simulink model "Pacemaker_OperatingModes"  (R2020a)
settings: Solver=FixedStepAuto  StartTime=0.0  StopTime=10.0  FixedStep=1e-3  RelTol=1e-3  EnableMultiTasking=on
undefined symbols (not defined in the file): D0, D1, D10, D11, D12, D13, D2, D3, D4, D5, D6, D7, D8, D9, PTA0, PTA1, PTA2, PTB23, PTB9, PTC16, PTC17, PTC2, PTC3, PTC4, PTD0, PTD1, PTD2, PTD3
libraries: frdmk64flib x14
settings Model: ExtModeTrigDuration=5  Creator=furqa  LastModifiedBy=furqa
settings OptimizationCC: EnhancedBackFolding=on  PassReuseOutputArgsAs=Individual arguments  ZeroExternalMemoryAtStartup=off  ZeroInternalMemoryAtStartup=off  MaxStackSize=64  OptimizeBlockOrder=speed  DifferentSizesBufferReuse=on  OptimizationCustomize=off  EfficientTunableParamExpr=on
settings DebuggingCC: ParameterTunabilityLossMsg=error
settings HardwareCC: ProdBitPerPointer=32  ProdBitPerSizeT=32  ProdBitPerPtrDiffT=32  ProdLargestAtomicInteger=Long  ProdLargestAtomicFloat=Double  ProdWordSize=32  ProdHWDeviceType=ARM Compatible->ARM Cortex
settings SFSimCC: MATLABDynamicMemAlloc=off
settings RTWCC: SystemTargetFile=ert.tlc  HardwareBoard=NXP FRDM-K64F  TemplateMakefile=ert_default_tmf  Toolchain=GNU Tools for ARM Embedded Processors
settings CodeAppCC: ForceParamTrailComments=on  IgnoreCustomStorageClasses=off  OperatorAnnotations=on  SimulinkDataObjDesc=on  SFDataObjDesc=on  InsertBlockDesc=on

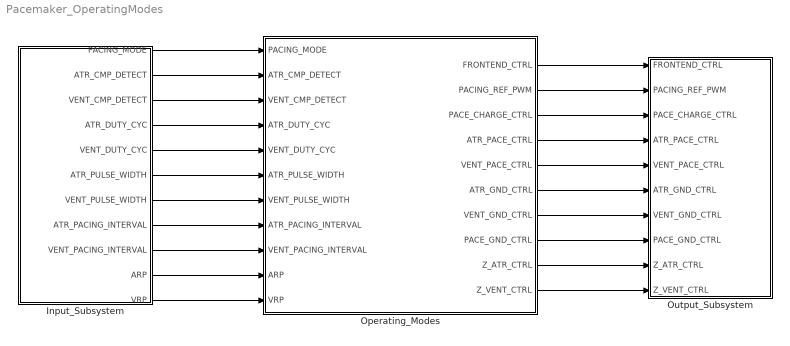
== system Pacemaker_OperatingModes ==
  Input_Subsystem : Subsystem
  Operating_Modes : Stateflow chart  TreatAsAtomicUnit=on
  Output_Subsystem : Subsystem
  wires:
  Input_Subsystem/1(PACING_MODE) -> Operating_Modes/1(PACING_MODE)
  Input_Subsystem/4(ATR_DUTY_CYC) -> Operating_Modes/4(ATR_DUTY_CYC)
  Input_Subsystem/5(VENT_DUTY_CYC) -> Operating_Modes/5(VENT_DUTY_CYC)
  Input_Subsystem/6("ATR_PULSE_WIDTH ") -> Operating_Modes/6(ATR_PULSE_WIDTH)
  Input_Subsystem/7("VENT_PULSE_WIDTH ") -> Operating_Modes/7(VENT_PULSE_WIDTH)
  Input_Subsystem/8("ATR_PACING_INTERVAL ") -> Operating_Modes/8(ATR_PACING_INTERVAL)
  Input_Subsystem/9("VENT_PACING_INTERVAL ") -> Operating_Modes/9(VENT_PACING_INTERVAL)
  Operating_Modes/1(FRONTEND_CTRL) -> Output_Subsystem/1(FRONTEND_CTRL)
  Operating_Modes/2(PACING_REF_PWM) -> Output_Subsystem/2(PACING_REF_PWM)
  Operating_Modes/3(PACE_CHARGE_CTRL) -> Output_Subsystem/3(PACE_CHARGE_CTRL)
  Operating_Modes/4(ATR_PACE_CTRL) -> Output_Subsystem/4(ATR_PACE_CTRL)
  Operating_Modes/5(VENT_PACE_CTRL) -> Output_Subsystem/5(VENT_PACE_CTRL)
  Operating_Modes/6(ATR_GND_CTRL) -> Output_Subsystem/6(ATR_GND_CTRL)
  Operating_Modes/7(VENT_GND_CTRL) -> Output_Subsystem/7(VENT_GND_CTRL)
  Operating_Modes/8(PACE_GND_CTRL) -> Output_Subsystem/8(PACE_GND_CTRL)
  Operating_Modes/9(Z_ATR_CTRL) -> Output_Subsystem/9(Z_ATR_CTRL)
  Operating_Modes/10(Z_VENT_CTRL) -> Output_Subsystem/10(Z_VENT_CTRL)
  Input_Subsystem/2(ATR_CMP_DETECT) -> Operating_Modes/2(ATR_CMP_DETECT)
  Input_Subsystem/3(VENT_CMP_DETECT) -> Operating_Modes/3(VENT_CMP_DETECT)
  Input_Subsystem/10(ARP) -> Operating_Modes/10(ARP)
  Input_Subsystem/11(VRP) -> Operating_Modes/11(VRP)

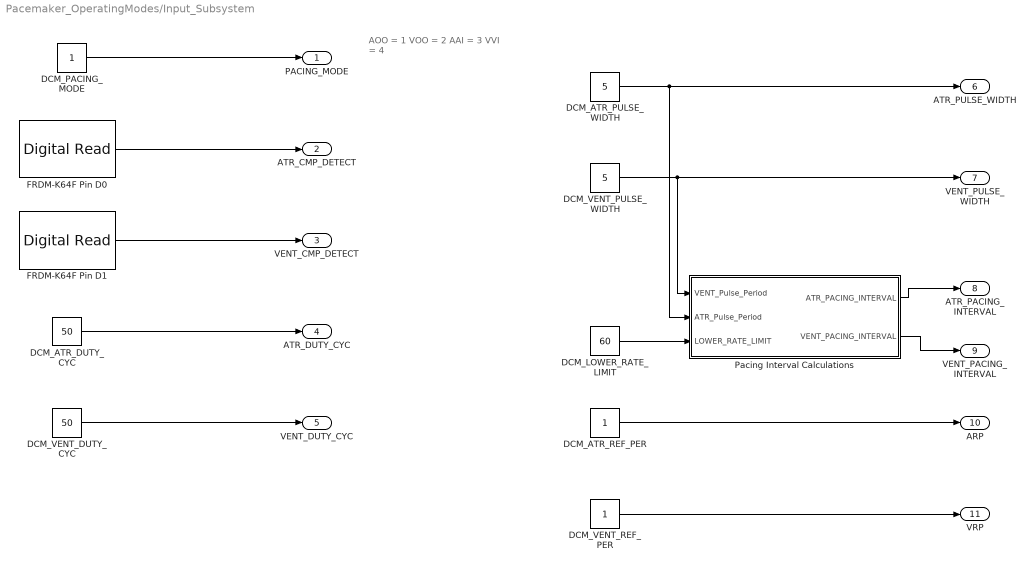
== system Pacemaker_OperatingModes/Input_Subsystem ==
  note: AOO = 1
      | VOO = 2
      | AAI = 3
      | VVI = 4
  DCM_ATR_DUTY_CYC : Constant  Value=50
  "DCM_ATR_PULSE_WIDTH " : Constant  Value=5
  DCM_ATR_REF_PER : Constant
  DCM_LOWER_RATE_LIMIT : Constant  Value=60
  DCM_PACING_MODE : Constant
  DCM_VENT_DUTY_CYC : Constant  Value=50
  "DCM_VENT_PULSE_WIDTH " : Constant  Value=5
  DCM_VENT_REF_PER : Constant
  FRDM-K64F Pin D0 : frdmk64flib/Digital Read  Whichpin=PTC16 (D0)  SampleTime=-1
  FRDM-K64F Pin D1 : frdmk64flib/Digital Read  Whichpin=PTC17 (D1)  SampleTime=-1
  Pacing Interval Calculations : Subsystem
  PACING_MODE : Outport
  ATR_CMP_DETECT : Outport  Port=2
  VENT_CMP_DETECT : Outport  Port=3
  ATR_DUTY_CYC : Outport  Port=4
  VENT_DUTY_CYC : Outport  Port=5
  "ATR_PULSE_WIDTH " : Outport  Port=6
  "VENT_PULSE_WIDTH " : Outport  Port=7
  "ATR_PACING_INTERVAL " : Outport  Port=8
  "VENT_PACING_INTERVAL " : Outport  Port=9
  ARP : Outport  Port=10
  VRP : Outport  Port=11
  wires:
  DCM_PACING_MODE/1 -> PACING_MODE/1
  FRDM-K64F Pin D0/1 -> ATR_CMP_DETECT/1
  FRDM-K64F Pin D1/1 -> VENT_CMP_DETECT/1
  DCM_ATR_DUTY_CYC/1 -> ATR_DUTY_CYC/1
  DCM_VENT_DUTY_CYC/1 -> VENT_DUTY_CYC/1
  "DCM_ATR_PULSE_WIDTH "/1 -> Pacing Interval Calculations/2(ATR_Pulse_Period), "ATR_PULSE_WIDTH "/1
  "DCM_VENT_PULSE_WIDTH "/1 -> "VENT_PULSE_WIDTH "/1, Pacing Interval Calculations/1(VENT_Pulse_Period)
  DCM_LOWER_RATE_LIMIT/1 -> Pacing Interval Calculations/3(LOWER_RATE_LIMIT)
  Pacing Interval Calculations/1(ATR_PACING_INTERVAL) -> "ATR_PACING_INTERVAL "/1
  Pacing Interval Calculations/2(VENT_PACING_INTERVAL) -> "VENT_PACING_INTERVAL "/1
  DCM_ATR_REF_PER/1 -> ARP/1
  DCM_VENT_REF_PER/1 -> VRP/1

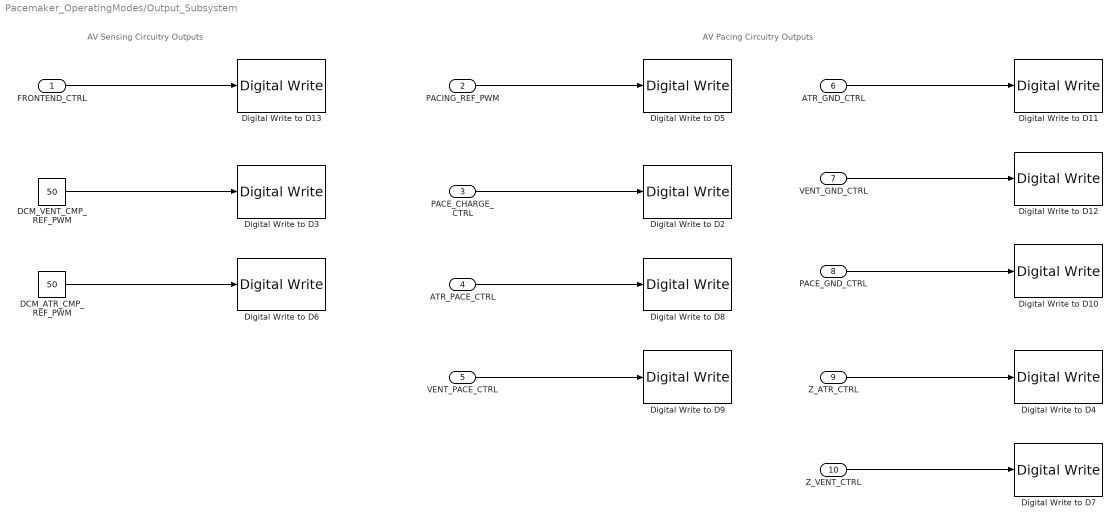
== system Pacemaker_OperatingModes/Output_Subsystem ==
  note: AV Pacing Circuitry Outputs
  note: AV Sensing Circuitry Outputs
  FRONTEND_CTRL : Inport
  PACING_REF_PWM : Inport  Port=2
  PACE_CHARGE_CTRL : Inport  Port=3
  ATR_PACE_CTRL : Inport  Port=4
  VENT_PACE_CTRL : Inport  Port=5
  ATR_GND_CTRL : Inport  Port=6
  VENT_GND_CTRL : Inport  Port=7
  PACE_GND_CTRL : Inport  Port=8
  Z_ATR_CTRL : Inport  Port=9
  Z_VENT_CTRL : Inport  Port=10
  DCM_ATR_CMP_REF_PWM : Constant  Value=50
  DCM_VENT_CMP_REF_PWM : Constant  Value=50
  Digital Write to D10 : frdmk64flib/Digital Write  Whichpin=PTD0 (D10)
  Digital Write to D11 : frdmk64flib/Digital Write  Whichpin=PTD2 (D11)
  Digital Write to D12 : frdmk64flib/Digital Write  Whichpin=PTD3 (D12)
  Digital Write to D13 : frdmk64flib/Digital Write  Whichpin=PTD1 (D13)
  Digital Write to D2 : frdmk64flib/Digital Write  Whichpin=PTB9 (D2)
  Digital Write to D3 : frdmk64flib/Digital Write  Whichpin=PTA1 (D3)
  Digital Write to D4 : frdmk64flib/Digital Write  Whichpin=PTB23 (D4)
  Digital Write to D5 : frdmk64flib/Digital Write  Whichpin=PTA2 (D5)
  Digital Write to D6 : frdmk64flib/Digital Write  Whichpin=PTC2 (D6)
  Digital Write to D7 : frdmk64flib/Digital Write  Whichpin=PTC3 (D7)
  Digital Write to D8 : frdmk64flib/Digital Write  Whichpin=PTA0 (D8)
  Digital Write to D9 : frdmk64flib/Digital Write  Whichpin=PTC4 (D9)
  wires:
  FRONTEND_CTRL/1 -> Digital Write to D13/1
  DCM_VENT_CMP_REF_PWM/1 -> Digital Write to D3/1
  DCM_ATR_CMP_REF_PWM/1 -> Digital Write to D6/1
  PACING_REF_PWM/1 -> Digital Write to D5/1
  PACE_CHARGE_CTRL/1 -> Digital Write to D2/1
  ATR_PACE_CTRL/1 -> Digital Write to D8/1
  VENT_GND_CTRL/1 -> Digital Write to D12/1
  VENT_PACE_CTRL/1 -> Digital Write to D9/1
  ATR_GND_CTRL/1 -> Digital Write to D11/1
  PACE_GND_CTRL/1 -> Digital Write to D10/1
  Z_ATR_CTRL/1 -> Digital Write to D4/1
  Z_VENT_CTRL/1 -> Digital Write to D7/1

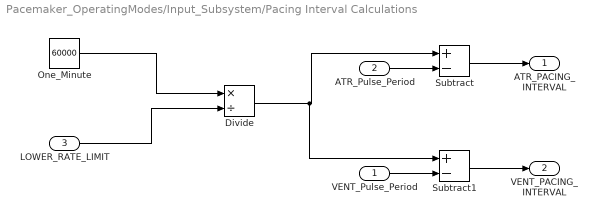
== system Pacemaker_OperatingModes/Input_Subsystem/Pacing Interval Calculations ==
  VENT_Pulse_Period : Inport
  ATR_Pulse_Period : Inport  Port=2
  LOWER_RATE_LIMIT : Inport  Port=3
  Divide : Product  Inputs=*/
  One_Minute : Constant  Value=60000
  Subtract : Sum  Inputs=+-
  Subtract1 : Sum  Inputs=+-
  ATR_PACING_INTERVAL : Outport
  VENT_PACING_INTERVAL : Outport  Port=2
  wires:
  One_Minute/1 -> Divide/1
  LOWER_RATE_LIMIT/1 -> Divide/2
  ATR_Pulse_Period/1 -> Subtract/2
  Subtract/1 -> ATR_PACING_INTERVAL/1
  VENT_Pulse_Period/1 -> Subtract1/2
  Divide/1 -> Subtract1/1, Subtract/1
  Subtract1/1 -> VENT_PACING_INTERVAL/1

== stateflow chart Pacemaker_OperatingModes/Operating_Modes ==
  state AOO
    state AOO_Pace_OFF
      during:
      ATR_PACE_CTRL = false
      VENT_PACE_CTRL = false
      PACING_REF_PWM = ATR_DUTY_CYC
      PACE_CHARGE_CTRL = true
      PACE_GND_CTRL = true
      Z_ATR_CTRL = false
      Z_VENT_CTRL = false
      ATR_GND_CTRL = true
      VENT_GND_CTRL = false
      FRONTEND_CTRL = false
    state AOO_Pace_ON
      during:
      PACE_CHARGE_CTRL = false
      PACE_GND_CTRL = true
      ATR_PACE_CTRL = true
      ATR_GND_CTRL = false
      Z_ATR_CTRL = false
      Z_VENT_CTRL = false
      VENT_GND_CTRL = false
      VENT_PACE_CTRL = false
      FRONTEND_CTRL = false
    (default) -> AOO_Pace_OFF
    AOO_Pace_OFF -> AOO_Pace_ON : after(ATR_PACING_INTERVAL, msec)
    AOO_Pace_ON -> AOO_Pace_OFF : after(ATR_PULSE_WIDTH, msec)
  state VVI
    state VVI_Pace_OFF
      during:
      ATR_PACE_CTRL = false
      VENT_PACE_CTRL = false
      PACING_REF_PWM =  VENT_DUTY_CYC
      PACE_CHARGE_CTRL = true
      PACE_GND_CTRL = true
      Z_ATR_CTRL = false
      Z_VENT_CTRL = false
      ATR_GND_CTRL = false
      VENT_GND_CTRL = true
      FRONTEND_CTRL = true
    state VVI_Pace_SENSED
      during:
      ATR_PACE_CTRL = false
      VENT_PACE_CTRL = false
      PACE_CHARGE_CTRL = true
      PACE_GND_CTRL = true
      Z_ATR_CTRL = false
      Z_VENT_CTRL = false
      ATR_GND_CTRL = false
      VENT_GND_CTRL = true
      FRONTEND_CTRL = false
    state VVI_Pace_ON
      during:
      PACE_CHARGE_CTRL = false
      PACE_GND_CTRL = true
      ATR_PACE_CTRL = false
      ATR_GND_CTRL = false
      Z_ATR_CTRL = false
      Z_VENT_CTRL = false
      VENT_GND_CTRL = false
      VENT_PACE_CTRL = true
      FRONTEND_CTRL = false
    VVI_Pace_ON -> VVI_Pace_OFF : after(VENT_PULSE_WIDTH , msec)
    (default) -> VVI_Pace_OFF
    VVI_Pace_OFF -> VVI_Pace_SENSED [order 1] : [VENT_CMP_DETECT==true]
    VVI_Pace_SENSED -> VVI_Pace_OFF : after(VRP,msec)
    VVI_Pace_OFF -> VVI_Pace_ON [order 2] : after(VENT_PACING_INTERVAL, msec)
  state VOO
    state VOO_Pace_OFF
      during:
      ATR_PACE_CTRL = false
      VENT_PACE_CTRL = false
      PACING_REF_PWM =  VENT_DUTY_CYC
      PACE_CHARGE_CTRL = true
      PACE_GND_CTRL = true
      Z_ATR_CTRL = false
      Z_VENT_CTRL = false
      ATR_GND_CTRL = false
      VENT_GND_CTRL = true
      FRONTEND_CTRL = false
    state VOO_Pace_ON
      during:
      PACE_CHARGE_CTRL = false
      PACE_GND_CTRL = true
      ATR_PACE_CTRL = false
      ATR_GND_CTRL = false
      Z_ATR_CTRL = false
      Z_VENT_CTRL = false
      VENT_GND_CTRL = false
      VENT_PACE_CTRL = true
      FRONTEND_CTRL = false
    (default) -> VOO_Pace_OFF
    VOO_Pace_OFF -> VOO_Pace_ON : after(VENT_PACING_INTERVAL, msec)
    VOO_Pace_ON -> VOO_Pace_OFF : after(VENT_PULSE_WIDTH , msec)
  state Start
  state AAI
    state AAI_Pace_OFF
      during:
      ATR_PACE_CTRL= false
      VENT_PACE_CTRL= false
      PACING_REF_PWM= ATR_DUTY_CYC
      PACE_CHARGE_CTRL= true
      PACE_GND_CTRL= true
      Z_ATR_CTRL= false
      Z_VENT_CTRL= false
      ATR_GND_CTRL= true
      VENT_GND_CTRL= false
      FRONTEND_CTRL= true
    state AAI_Pace_ON
      during:
      PACE_CHARGE_CTRL= false
      PACE_GND_CTRL= true
      ATR_PACE_CTRL= true
      ATR_GND_CTRL= false
      Z_ATR_CTRL= false
      Z_VENT_CTRL= false
      VENT_GND_CTRL= false
      VENT_PACE_CTRL= false
      FRONTEND_CTRL= false
    state AAI_Pace_SENSED
      during:
      ATR_PACE_CTRL= false
      VENT_PACE_CTRL= false
      PACE_CHARGE_CTRL= true
      PACE_GND_CTRL= true
      Z_ATR_CTRL= false
      Z_VENT_CTRL= false
      ATR_GND_CTRL= true
      VENT_GND_CTRL= false
      FRONTEND_CTRL= false
    AAI_Pace_ON -> AAI_Pace_OFF : after(ATR_PULSE_WIDTH,msec)
    (default) -> AAI_Pace_OFF
    AAI_Pace_OFF -> AAI_Pace_SENSED [order 2] : [ATR_CMP_DETECT==true]
    AAI_Pace_SENSED -> AAI_Pace_OFF : after(ARP,msec)
    AAI_Pace_OFF -> AAI_Pace_ON [order 1] : after(ATR_PACING_INTERVAL,msec)
  Start -> AOO [order 1] : [PACING_MODE == 1]
  AOO -> Start : [PACING_MODE ~= 1]
  (default) -> Start
  Start -> VVI [order 4] : [PACING_MODE == 4]
  Start -> VOO [order 2] : [PACING_MODE == 2]
  VOO -> Start : [PACING_MODE~=2]
  VVI -> Start : [PACING_MODE~=4]
  Start -> AAI [order 3] : [PACING_MODE == 3]
  AAI -> Start : [PACING_MODE~=3]
  data: FRONTEND_CTRL output; PACING_REF_PWM output; PACE_CHARGE_CTRL output; ATR_PACE_CTRL output; VENT_PACE_CTRL output; ATR_GND_CTRL output; VENT_GND_CTRL output; PACE_GND_CTRL output; Z_ATR_CTRL output; Z_VENT_CTRL output; PACING_MODE input; ATR_CMP_DETECT input; VENT_CMP_DETECT input; ATR_DUTY_CYC input; VENT_DUTY_CYC input; ATR_PULSE_WIDTH input; VENT_PULSE_WIDTH input; ATR_PACING_INTERVAL input; VENT_PACING_INTERVAL input; ARP input; VRP input
